simulink model "Smart_City_QCar2_self_driving_stack"  (R2024b)
settings: Solver=ode1  StartTime=0.0  StopTime=inf  FixedStep=Controller_Sample_Time  RelTol=1e-3  EnableMultiTasking=on
values from neighbouring files (symbols this model uses):
  angles_qcar2 = angles_new_qcar2(2: length (angles_new_qcar2), width (angles_new_qcar2)-5)    [Setup_QCar1and2_params.m]
  Audio_Sample_Time = 0.3    [Setup_QCar1and2_params.m]
  cal_pos = [0, 0, 0]    [Setup_QCar1and2_params.m]
  cameraStepSize = 3e-2    (= 0.03)    [Setup_QCar1and2_params.m]
  Cobra_Start = [0 0 0 0 0 0 0 0 0 0 0 0 ... (192000 elements, 192000x1)]    [QCar_Sounds.mat]
  Controller_Sample_Time = CSI_Sample_Time/10    (= 0.00166666666667)    [Setup_QCar1and2_params.m]
  CSI_Sample_Time = 1/60    (= 0.0166666666667)    [Setup_QCar1and2_params.m]
  engine = [0.455749511719 0.619506835938 0.612854003906 0.499603271484 0.347473144531 0.278045654297 0.304656982422 0.258544921875 0.100128173828 0.0902099609375 0.341461181641 0.515716552734 ... (88200 elements, 44100x2)]    [QCar_Sounds.mat]
  GyroKF_P0 = eye(2)    [Setup_QCar1and2_params.m]
  GyroKF_Q = diag([0.01, 0.001])    [Setup_QCar1and2_params.m]
  GyroKF_R = 0.01    [Setup_QCar1and2_params.m]
  GyroKF_X0 = [0;0]    [Setup_QCar1and2_params.m]
  honk = [0.01708984375 0.0179443359375 0.018798828125 0.019775390625 0.0209655761719 0.0218505859375 0.0221557617188 0.0223693847656 0.022705078125 0.023681640625 0.0252075195312 0.0257263183594 ... (43568 elements, 21784x2)]    [QCar_Sounds.mat]
  ImageDisplay_Sample_Time = CSI_Sample_Time*6    (= 0.1)    [Setup_QCar1and2_params.m]
  Initialization_Time = 5    [Setup_QCar1and2_params.m]
  LiDAR_Sample_Time = CSI_Sample_Time*3    (= 0.05)    [Setup_QCar1and2_params.m]
  map_mask = [1 1 1 0 0 1 0]    [Setup_QCar1and2_params.m]
  NN_Sample_Time = RealSense_Sample_Time*1    (= 0.0333333333333)    [Setup_QCar1and2_params.m]
  path_x = [0.826 0.836 0.846 0.856 0.866 0.876 0.886 0.896 0.906 0.916 0.926 0.936 ... (740 elements, 740x1)]    [SDCS_Paths_7.mat]
  path_x2 = [-0.614 -0.604 -0.594 -0.584 -0.574 -0.564 -0.554 -0.544 -0.534 -0.524 -0.514 -0.504 ... (1090 elements, 1090x1)]    [SDCS_Paths_7.mat]
  path_x3 = [-0.614 -0.603821428571 -0.593642857143 -0.583464285714 -0.573285714286 -0.563107142857 -0.552928571429 -0.54275 -0.532571428571 -0.522392857143 -0.512214285714 -0.502035714286 ... (714 elements, 714x1)]    [SDCS_Paths_7.mat]
  path_x4 = [-0.614 -0.604 -0.594 -0.584 -0.574 -0.564 -0.554 -0.544 -0.534 -0.524 -0.514 -0.504 ... (1761 elements, 1761x1)]    [SDCS_Paths_7.mat]
  path_x5 = [1.436 1.42588571429 1.41577142857 1.40565714286 1.39554285714 1.38542857143 1.37531428571 1.3652 1.35508571429 1.34497142857 1.33485714286 1.32474285714 ... (574 elements, 574x1)]    [SDCS_Paths_7.mat]
  path_x6 = [1.436 1.42588571429 1.41577142857 1.40565714286 1.39554285714 1.38542857143 1.37531428571 1.3652 1.35508571429 1.34497142857 1.33485714286 1.32474285714 ... (1288 elements, 1288x1)]    [SDCS_Paths_7.mat]
  path_x7 = [-1.5778487585 -1.56959877056 -1.56127865467 -1.55288878259 -1.54442952915 -1.53590127231 -1.52730439309 -1.51863927561 -1.50990630701 -1.50110587746 -1.49223838016 -1.4833042113 ... (2260 elements, 2260x1)]    [SDCS_Paths_7.mat]
  path_y = [-1.0887 -1.0887 -1.0887 -1.0887 -1.0887 -1.0887 -1.0887 -1.0887 -1.0887 -1.0887 -1.0887 -1.0887 ... (740 elements, 740x1)]    [SDCS_Paths_7.mat]
  path_y2 = [-1.0887 -1.0887 -1.0887 -1.0887 -1.0887 -1.0887 -1.0887 -1.0887 -1.0887 -1.0887 -1.0887 -1.0887 ... (1090 elements, 1090x1)]    [SDCS_Paths_7.mat]
  path_y3 = [-1.0887 -1.0887 -1.0887 -1.0887 -1.0887 -1.0887 -1.0887 -1.0887 -1.0887 -1.0887 -1.0887 -1.0887 ... (714 elements, 714x1)]    [SDCS_Paths_7.mat]
  path_y4 = [-1.0887 -1.0887 -1.0887 -1.0887 -1.0887 -1.0887 -1.0887 -1.0887 -1.0887 -1.0887 -1.0887 -1.0887 ... (1761 elements, 1761x1)]    [SDCS_Paths_7.mat]
  path_y5 = [-0.8157 -0.8157 -0.8157 -0.8157 -0.8157 -0.8157 -0.8157 -0.8157 -0.8157 -0.8157 -0.8157 -0.8157 ... (574 elements, 574x1)]    [SDCS_Paths_7.mat]
  path_y6 = [-0.8157 -0.8157 -0.8157 -0.8157 -0.8157 -0.8157 -0.8157 -0.8157 -0.8157 -0.8157 -0.8157 -0.8157 ... (1288 elements, 1288x1)]    [SDCS_Paths_7.mat]
  path_y7 = [-0.614490295955 -0.61974988896 -0.624981792226 -0.630185771997 -0.635361595765 -0.640509032279 -0.645627851559 -0.6507178249 -0.655778724888 -0.660810325409 -0.665812401655 -0.670784730139 ... (2260 elements, 2260x1)]    [SDCS_Paths_7.mat]
  put_me_down = [0 0 0 0 0 0 0 0 0 0 0 0 ... (335870 elements, 167935x2)]    [QCar_Sounds.mat]
  qcar2_lidar_to_map_rotation = 0    [Setup_QCar1and2_params.m]
  QCarEKF_L = 0.24    [Setup_QCar1and2_params.m]
  QCarEKF_P0 = eye(3)    [Setup_QCar1and2_params.m]
  QCarEKF_Q = diag([0.00001, 0.00001, 0.00001])    [Setup_QCar1and2_params.m]
  QCarEKF_R_combined = diag([0.1, 0.1, 0.01])    [Setup_QCar1and2_params.m]
  QCarEKF_R_heading = diag(0.1)    [Setup_QCar1and2_params.m]
  QcarKF_X0 = [0; 0; 0]    [Setup_QCar1and2_params.m]
  range_qcar2 = distance_new_qcar2(2: length (distance_new_qcar2), width (distance_new_qcar2)-5)    [Setup_QCar1and2_params.m]
  RealSense_Sample_Time = CSI_Sample_Time*2    (= 0.0333333333333)    [Setup_QCar1and2_params.m]
  truck_start = [0.00137329101562 0.00115966796875 0.0006103515625 0.000762939453125 0.00115966796875 0.00198364257812 0.00115966796875 0.000762939453125 0.00137329101562 0.00115966796875 0.00115966796875 0.000762939453125 ... (60000 elements, 60000x1)]    [QCar_Sounds.mat]
undefined symbols (not defined in the file or in its folder): DiscIntNeverNeededParam, gcbh, height, HIL, Joystick_Sample_Time, JPEG, left, Point, qc_get_step_size, top, video_display_show, width
libraries: quarc_library x65, simulink_extras x12, simulink x8
(part 3 of 5)

== system Smart_City_QCar2_self_driving_stack/QCar 2/QCar Control/QCar I//O ==
  note: '-w -d /tmp -uri %u', 'tcpip://192.168.1.3:17002'
  note: Command Conditioning
  note: HIL I/O
  note: LEDs:
      | 1. Back Left Amber
      | 2. Back Right Amber
      | 3. Front Left Amber
      | 4. Front Right Amber
      | 5. Brake Lights Red
      | 6. Reverse White
      | 7. Left Headlamps White
      | 8. Right Headlamps White
  "motorCmd (%, rad) [2]" : Inport
  Arm : Inport  Port=2
  Hazard : Inport  Port=3
  Volume : Inport  Port=4
  Honk : Inport  Port=5
  Abs : Abs  SaturateOnIntegerOverflow=off
  Audio : Subsystem
  Constant1 : Constant
  Constant3 : Constant  Value=.05
  Constant4 : Constant  Value=.05
  Constant6 : Constant  Value=2
  Demux : Demux  Outputs=2
  Display : Display
  Gain : Gain  Gain=+1
  Greater Than Threshold : Subsystem
  HIL Initialize : quarc_library/Data Acquisition/Generic/Configuration/HIL Initialize  object_name=HIL-1  board_type=qcar2  board_number=0  board_options=gyro_fs=250;gyro_rate=500;gyro_bw=125;gyro_ord=3;accel_fs=16;accel_rate=1000;accel_bw=250;accel_ord=3;temp_bw=4000;enc0_dir=0;enc1_dir=0;enc2_dir=0;steer_bias=0.05;  exclusive=off  active=on  hardware_clocks=[]  clock_modes=[]  initial_clock_frequencies=[]  set_clock_params_at_start=off  set_clock_params_at_switch_in=off  set_clock_frequencies_at_start=off  set_clock_frequencies_at_switch_in=off  analog_input_channels=[0:4]  analog_input_configurations=[]  analog_input_maximums=[3.3]  analog_input_minimums=[0]  set_analog_input_params_at_start=off  set_analog_input_params_at_switch_in=off  analog_output_channels=[]  analog_output_maximums=[]  analog_output_minimums=[]  initial_analog_outputs=[]  final_analog_outputs=[]  watchdog_analog_outputs=[]  set_analog_output_params_at_start=off  set_analog_output_params_at_switch_in=off  set_analog_outputs_at_start=off  set_analog_outputs_at_switch_in=off  set_analog_outputs_at_terminate=off  set_analog_outputs_at_switch_out=off  set_analog_outputs_on_watchdog=off  digital_input_channels=[0:14]  digital_output_channels=[11:26]  digital_output_configuration=[]  initial_digital_outputs=[0]  final_digital_outputs=[0]  watchdog_digital_outputs=[0]  set_digital_output_params_at_start=off  set_digital_output_params_at_switch_in=off  set_digital_outputs_at_start=on  set_digital_outputs_at_switch_in=off  set_digital_outputs_at_terminate=on  set_digital_outputs_at_switch_out=off  set_digital_outputs_on_watchdog=off  encoder_channels=[0:2]  quadrature=[4]  encoder_filter_frequency=100e6/1  initial_encoder_counts=[0]  set_encoder_params_at_start=on  set_encoder_params_at_switch_in=off  set_encoder_counts_at_start=on  set_encoder_counts_at_switch_in=off  pwm_channels=[0:1]  pwm_modes=[0]  pwm_frequency=180e6/4096  pwm_configuration=[0]  pwm_alignment=[0]  pwm_polarity=[1]  pwm_leading_deadband=[]  pwm_trailing_deadband=[]  initial_pwm_outputs=[0]  final_pwm_outputs=[0]  watchdog_pwm_outputs=[0]  set_pwm_params_at_start=on  set_pwm_params_at_switch_in=off  set_pwm_outputs_at_start=on  set_pwm_outputs_at_switch_in=off  set_pwm_outputs_at_terminate=on  set_pwm_outputs_at_switch_out=off  set_pwm_outputs_on_watchdog=off  other_output_channels=[1000 11000]  initial_other_outputs=[0]  final_other_outputs=[0]  watchdog_other_outputs=[0]  set_other_outputs_at_start=on  set_other_outputs_at_switch_in=off  set_other_outputs_at_terminate=on  set_other_outputs_at_switch_out=off  set_other_outputs_on_watchdog=off
  HIL Read : quarc_library/Data Acquisition/Generic/Immediate I//O/HIL Read  object_name=HIL-1  analog_channels=[4 2]  encoder_channels=[0]  digital_channels=[]  other_channels=[14000 3002 4001]  sample_time=qc_get_step_size  active=on  vector_output=off  data_type_mode=Inherit via back propagation  encoder_data_type=double  digital_data_type=boolean
  HIL Write : quarc_library/Data Acquisition/Generic/Immediate I//O/HIL Write  object_name=HIL-1  analog_channels=[]  pwm_channels=[]  digital_channels=[17:18 25:26 11:16 19:24]  other_channels=[1000 11000]  sample_time=-1  active=off  vector_input=on
  LEDs : Subsystem
  Less Than Threshold1 : Subsystem
  MATLAB Function : MATLAB Function  TreatAsAtomicUnit=on
  Memory : Memory
  Mux : Mux  Inputs=2
  Scope : Scope
  Steering Bias : Bias  Bias=0.05*-1  SaturateOnIntegerOverflow=off
  Unwrap 2^24 : quarc_library/Discontinuities/Inverse Modulus  modulus=16777215  output_derivative=off  output_revolutions=off  max_x=Inf  min_x=-Inf
  basicSpeedEstimation : Subsystem
  basicSpeedEstimation1 : Subsystem
  command saturation : Saturate  UpperLimit=.6  LowerLimit=-0.6
  direction convention : Gain  Gain=+1
  motorCurrent (A) [1] : Outport  VectorParamsAs1DForOutWhenUnconnected=off
  batteryVoltage (V) [1] : Outport  Port=2  VectorParamsAs1DForOutWhenUnconnected=off
  Speed (m/s) : Outport  Port=3  VectorParamsAs1DForOutWhenUnconnected=off
  gyroscopicRates (rad/s) : Outport  Port=4  VectorParamsAs1DForOutWhenUnconnected=off
  Odometer : Outport  Port=5  VectorParamsAs1DForOutWhenUnconnected=off
  wires:
  Demux/2 -> MATLAB Function/1(steering_in), LEDs/2(Steering)
  direction convention/1 -> command saturation/1
  "motorCmd (%, rad) [2]"/1 -> Demux/1
  HIL Read/3 -> Unwrap 2^24/1  "encoder counts"
  Gain/1 -> Steering Bias/1
  HIL Read/1 -> motorCurrent (A) [1]/1  "motor current"
  HIL Read/2 -> batteryVoltage (V) [1]/1  "battery voltage"
  HIL Read/4 -> basicSpeedEstimation/1(motorSpeed (counts/s))
  Unwrap 2^24/1 -> basicSpeedEstimation1/1(motorSpeed (counts/s))
  basicSpeedEstimation1/1(longitudinalCarSpeed (m/s)) -> Odometer/1
  basicSpeedEstimation/1(longitudinalCarSpeed (m/s)) -> [Speed], Speed (m/s)/1
  Demux/1 -> LEDs/1(Throttle), Scope/1, direction convention/1
  HIL Read/5 -> gyroscopicRates (rad/s)/1
  LEDs/1(LEDs) -> HIL Write/1
  Honk/1 -> Audio/1(Honk)
  Arm/1 -> Audio/2(Arm)
  [Speed] -> LEDs/3(Speed)
  Hazard/1 -> LEDs/4(Hazzard)
  HIL Read/6 -> Abs/1
  Abs/1 -> Greater Than Threshold/1(Signal)
  Constant6/1 -> Greater Than Threshold/2(Threshold)
  Constant1/1 -> Greater Than Threshold/3(Duration)
  Greater Than Threshold/1(elapsed) -> Audio/3(put_me_down)
  Volume/1 -> Audio/4(Volume)
  Constant3/1 -> Less Than Threshold1/2(Threshold)
  Constant4/1 -> Less Than Threshold1/3(Duration)
  [Speed] -> Less Than Threshold1/1(Signal)
  MATLAB Function/1(steering_out) -> Gain/1, Memory/1
  Less Than Threshold1/1(elapsed) -> Display/1, MATLAB Function/2(stopped)
  Memory/1 -> MATLAB Function/3(previous_steering)
  Mux/1 -> HIL Write/2
  Steering Bias/1 -> Mux/1
  command saturation/1 -> Mux/2

== system Smart_City_QCar2_self_driving_stack/QCar 2/QCar Control/bicycleModel ==
  note: coordinate transformation
  note: Model side slip angle beta
  note: steering servo dynamics
  heading (rad) : Inport
  "motorCommands (%, rad)" : Inport  Port=2
  carSpeed (m/s) : Inport  Port=3
  gyroscope (rad/s) : Inport  Port=4
  Add : Sum
  Divide : Product  Inputs=*/
  Lr : Constant  Value=0.128
  Mux3 : Mux  Inputs=3
  Product : Product
  Product1 : Product
  Product2 : Product
  Transfer Fcn : TransferFcn  Denominator=[0.1026 1]
  Trigonometric Function : Trigonometry
  Trigonometric Function1 : Trigonometry  Operator=cos
  Trigonometric Function2 : Trigonometry  Operator=tan
  Trigonometric Function3 : Trigonometry  Operator=atan
  select steering : Selector  InputPortWidth=2  IndexOptions=Index vector (dialog)  Indices=[2]  OutputSizes=1
  steering servo dynamics : Scope  NumInputPorts=2
  wheelbase : Constant  Value=0.256
  "poseRate (m/s, m/s, rad/s)" : Outport  VectorParamsAs1DForOutWhenUnconnected=off
  wires:
  Add/1 -> Trigonometric Function1/1, Trigonometric Function/1
  Trigonometric Function1/1 -> Product1/2
  Product/1 -> Mux3/2  "y_dot"
  select steering/1 -> Transfer Fcn/1, steering servo dynamics/1  "delta"
  carSpeed (m/s)/1 -> Product/2, Product1/1  "v"
  Product1/1 -> Mux3/1  "x_dot"
  Trigonometric Function/1 -> Product/1
  gyroscope (rad/s)/1 -> Mux3/3  "psi_dot"
  heading (rad)/1 -> Add/1  "psi"
  "motorCommands (%, rad)"/1 -> select steering/1
  Mux3/1 -> "poseRate (m/s, m/s, rad/s)"/1
  Transfer Fcn/1 -> Trigonometric Function2/1, steering servo dynamics/2
  Divide/1 -> Trigonometric Function3/1
  wheelbase/1 -> Divide/2
  Product2/1 -> Divide/1  "Lr tan(delta)"
  Trigonometric Function3/1 -> Add/2  "beta"
  Trigonometric Function2/1 -> Product2/1  "tan(delta)"
  Lr/1 -> Product2/2  "Lr"

== system Smart_City_QCar2_self_driving_stack/QCar 2/QCar Control/powerConsumptionMonitor ==
  note: Battery percentage calculation
  note: P = VI
  note: Electrical
      | power
      | consumed
  note: Power Monitoring Module:
      |
      | This subsystem monitors power consumption and provides a percentage battery remaining indicator.
      |
      | Inputs:
      | motorCurrent (A) n/a : Motor current being pulled by the main drive motor
      | batteryVoltage (V) {0, 12.6} : Current battery voltage reading
      |
      | Outputs:
      | motorPowerConsumption (W) n/a : Current power in Watts being pulled by the main drive motor
      | batteryLevel (%) {0,1} : Percentage battery level remaining
      |
      | Usage:
      | This is based on a maximum 3S battery voltage of 12.6 V (4.2V per cell) and minimum of 10.5 V (3.5V per cell)
  motorCurrent (A) [1] : Inport
  batteryVoltage (V) [1] : Inport  Port=2
  Divide : Product  Inputs=*/
  Gain : Gain  Gain=100
  Product : Product
  Subtract : Sum  Inputs=+-
  Subtract1 : Sum  Inputs=+-
  max voltage : Constant  Value=12.6
  min voltage : Constant  Value=10.5
  motorPowerConsumption (W) [1] : Outport  VectorParamsAs1DForOutWhenUnconnected=off
  batteryLevel (%) [1] : Outport  Port=2  VectorParamsAs1DForOutWhenUnconnected=off
  wires:
  Divide/1 -> Gain/1
  Subtract1/1 -> Divide/2
  Gain/1 -> batteryLevel (%) [1]/1
  Product/1 -> motorPowerConsumption (W) [1]/1
  min voltage/1 -> Subtract/2, Subtract1/2
  motorCurrent (A) [1]/1 -> Product/1
  max voltage/1 -> Subtract1/1
  Subtract/1 -> Divide/1
  batteryVoltage (V) [1]/1 -> Subtract/1, Product/2

== system Smart_City_QCar2_self_driving_stack/QCar 2/QCar Control/speedController ==
  note: Feedforward
  note: Feedback
  arm (0,1) : Inport
  desiredSpeed (m/s) : Inport  Port=2
  measuredSpeed (m/s) : Inport  Port=3
  Add : Sum
  Add1 : Sum
  Compare To Zero : simulink/Logic and Bit Operations/Compare To Zero  relop===  OutDataTypeStr=boolean
  Demux : Demux  Outputs=2
  Integrator1 : Integrator  ExternalReset=either  LimitOutput=on  UpperSaturationLimit=0.4  LowerSaturationLimit=-0.4
  Kff (% / m/s) : Gain  Gain=0.1
  "Ki (% / m) " : Gain
  Kp (% / m/s) : Gain  Gain=.3
  Multiply : Product
  Multiply1 : Product
  Multiply2 : Product
  Mux : Mux  Inputs=2
  Speed_Tracking : Scope  NumInputPorts=2
  Sum : Sum  Inputs=|+-
  command saturation : Saturate  UpperLimit=5  LowerLimit=-5
  throttleCmd (%) : Outport  VectorParamsAs1DForOutWhenUnconnected=off
  wires:
  command saturation/1 -> Multiply1/1  "desired"
  arm (0,1)/1 -> Multiply1/2, Multiply/2, Multiply2/2
  measuredSpeed (m/s)/1 -> Multiply/1  "meas"
  Multiply/1 -> Sum/2, Speed_Tracking/2  "measured"
  Add/1 -> Add1/2
  Add1/1 -> Multiply2/1  "%"
  Multiply1/1 -> Compare To Zero/1, Sum/1, Kff (% / m/s)/1, Speed_Tracking/1  "desired"
  Integrator1/1 -> Add/2
  Kp (% / m/s)/1 -> Add/1
  Compare To Zero/1 -> Integrator1/2
  Kff (% / m/s)/1 -> Add1/1
  Sum/1 -> "Ki (% / m) "/1, Kp (% / m/s)/1
  "Ki (% / m) "/1 -> Integrator1/1
  Multiply2/1 -> Mux/1  "pwm duty cycle"
  Mux/1 -> throttleCmd (%)/1
  desiredSpeed (m/s)/1 -> Demux/1
  Demux/1 -> command saturation/1
  Demux/2 -> Mux/2

== system Smart_City_QCar2_self_driving_stack/QCar 2/QCar Control/turnSpeedHandling ==
  Commands in : Inport
  Cos ^ : Inport  Port=2
  Cos : Trigonometry  Operator=cos
  Demux1 : Demux  Outputs=2
  Mux : Mux  Inputs=2
  Product : Product
  Saturation : Saturate  UpperLimit=1  LowerLimit=.3
  Speed Comparison : Scope  NumInputPorts=2
  Square : Math  Operator=pow  SignedPower=on
  Commands : Outport  VectorParamsAs1DForOutWhenUnconnected=off
  wires:
  Cos/1 -> Square/1
  Saturation/1 -> Product/2
  Demux1/1 -> Product/1, Speed Comparison/1  "Input Speed"
  Commands in/1 -> Demux1/1
  Cos ^/1 -> Square/2
  Square/1 -> Saturation/1
  Product/1 -> Mux/1, Speed Comparison/2  "Ouput Speed"
  Mux/1 -> Commands/1
  Demux1/2 -> Mux/2, Cos/1  "input steering"

== system Smart_City_QCar2_self_driving_stack/Randomizer1/Subsystem1/RisingEdge ==
  Input : Inport
  Logical Operator1 : Logic  AllPortsSameDT=off
  Logical Operator2 : Logic  Operator=NOT  AllPortsSameDT=off
  Memory : Memory  InheritSampleTime=on  LinearizeMemory=on
  RisingEdgeTrigger : Outport  VectorParamsAs1DForOutWhenUnconnected=off
  wires:
  Logical Operator1/1 -> RisingEdgeTrigger/1
  Logical Operator2/1 -> Logical Operator1/2
  Memory/1 -> Logical Operator2/1
  Input/1 -> Logical Operator1/1, Memory/1

== system Smart_City_QCar2_self_driving_stack/Speed & Steering Commander/Path Commander/Less Than Threshold ==
  note: Calculate Duration that Car is in Distance of Viable Path
  Distances : Inport
  Distance Threshold : Inport  Port=2
  Duration Threshold : Inport  Port=3
  Data Type Conversion : DataTypeConversion  SaturateOnIntegerOverflow=off  RndMeth=Floor
  Discrete-Time Integrator : DiscreteIntegrator  Priority=1  ExternalReset=level  SampleTime=qc_get_step_size  ICPrevOutput=DiscIntNeverNeededParam  ICPrevScaledInput=DiscIntNeverNeededParam
  Relational Operator : RelationalOperator  Operator=<  InputSameDT=off
  Relational Operator1 : RelationalOperator  InputSameDT=off
  Reset Condition : Logic  Operator=NOT  AllPortsSameDT=off  OutDataTypeStr=boolean
  elapsed : Outport  VectorParamsAs1DForOutWhenUnconnected=off
  wires:
  Data Type Conversion/1 -> Discrete-Time Integrator/1
  Distances/1 -> Relational Operator/1
  Distance Threshold/1 -> Relational Operator/2
  Relational Operator/1 -> Data Type Conversion/1, Reset Condition/1
  Reset Condition/1 -> Discrete-Time Integrator/2
  Discrete-Time Integrator/1 -> Relational Operator1/1
  Duration Threshold/1 -> Relational Operator1/2
  Relational Operator1/1 -> elapsed/1

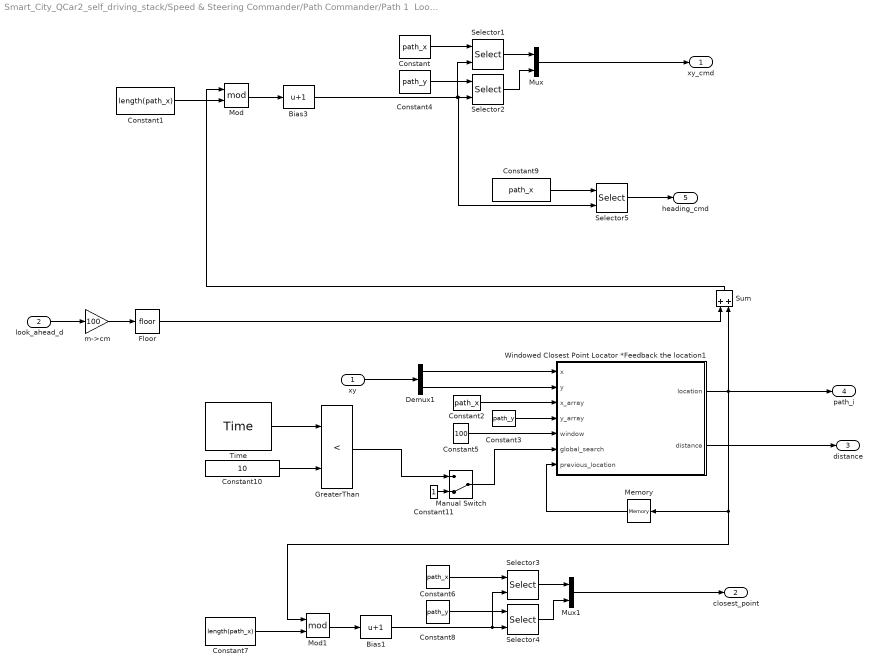
== system Smart_City_QCar2_self_driving_stack/Speed & Steering Commander/Path Commander/Path 1  Look Ahead Generator ==
  xy : Inport
  look_ahead_d : Inport  Port=2
  Bias1 : Bias  Bias=1  SaturateOnIntegerOverflow=off
  Bias3 : Bias  Bias=1  SaturateOnIntegerOverflow=off
  Constant{,2,6,9} (4 alike) : Constant  Value=path_x
  Constant1 : Constant  Value=length(path_x)
  Constant10 : Constant  Value=10
  Constant11 : Constant
  Constant3 : Constant  Value=path_y
  Constant4 : Constant  Value=path_y
  Constant5 : Constant  Value=100
  Constant7 : Constant  Value=length(path_x)
  Constant8 : Constant  Value=path_y
  Demux1 : Demux  Outputs=2
  Floor : Rounding
  GreaterThan : RelationalOperator  Operator=<  OutDataTypeStr=boolean  RndMeth=Simplest  InputSameDT=off
  Manual Switch : ManualSwitch  CurrentSetting=0
  Memory : Memory  InitialCondition=1  InheritSampleTime=on  LinearizeMemory=on  LinearizeAsDelay=on
  Mod : Math  Operator=mod
  Mod1 : Math  Operator=mod
  Mux : Mux  Inputs=2
  Mux1 : Mux  Inputs=2
  Selector{1..5} (5 alike) : Selector  InputPortWidth=length(path_x)  IndexOptions=Index vector (port)  Indices=[1 3]  OutputSizes=1
  Sum : Sum
  Time : quarc_library/Sources/Time/Time  time_source=Wall clock  sample_time=qc_get_step_size
  Windowed Closest Point Locator *Feedback the location1 : MATLAB Function  TreatAsAtomicUnit=on
  m->cm : Gain  Gain=100
  xy_cmd : Outport
  closest_point : Outport  Port=2
  distance : Outport  Port=3
  path_i : Outport  Port=4
  heading_cmd : Outport  Port=5
  wires:
  Demux1/1 -> Windowed Closest Point Locator *Feedback the location1/1(x)
  Constant2/1 -> Windowed Closest Point Locator *Feedback the location1/3(x_array)
  Constant3/1 -> Windowed Closest Point Locator *Feedback the location1/4(y_array)
  Constant1/1 -> Mod/2
  Sum/1 -> Mod/1
  Demux1/2 -> Windowed Closest Point Locator *Feedback the location1/2(y)
  Mod/1 -> Bias3/1
  xy/1 -> Demux1/1
  look_ahead_d/1 -> m->cm/1
  m->cm/1 -> Floor/1
  Floor/1 -> Sum/1
  Constant/1 -> Selector1/1
  Selector1/1 -> Mux/1
  Constant4/1 -> Selector2/1
  Mux/1 -> xy_cmd/1
  Selector2/1 -> Mux/2
  Windowed Closest Point Locator *Feedback the location1/2(distance) -> distance/1
  Mux1/1 -> closest_point/1
  Bias1/1 -> Selector3/2, Selector4/2
  Selector4/1 -> Mux1/2
  Constant6/1 -> Selector3/1
  Mod1/1 -> Bias1/1
  Constant7/1 -> Mod1/2
  Constant8/1 -> Selector4/1
  Selector3/1 -> Mux1/1
  Windowed Closest Point Locator *Feedback the location1/1(location) -> Sum/2, path_i/1, Mod1/1, Memory/1
  Bias3/1 -> Selector1/2, Selector5/2, Selector2/2
  Constant9/1 -> Selector5/1
  Selector5/1 -> heading_cmd/1
  Time/1 -> GreaterThan/1
  Constant10/1 -> GreaterThan/2
  Constant5/1 -> Windowed Closest Point Locator *Feedback the location1/5(window)
  Memory/1 -> Windowed Closest Point Locator *Feedback the location1/7(previous_location)
  Constant11/1 -> Manual Switch/2
  Manual Switch/1 -> Windowed Closest Point Locator *Feedback the location1/6(global_search)
  GreaterThan/1 -> Manual Switch/1

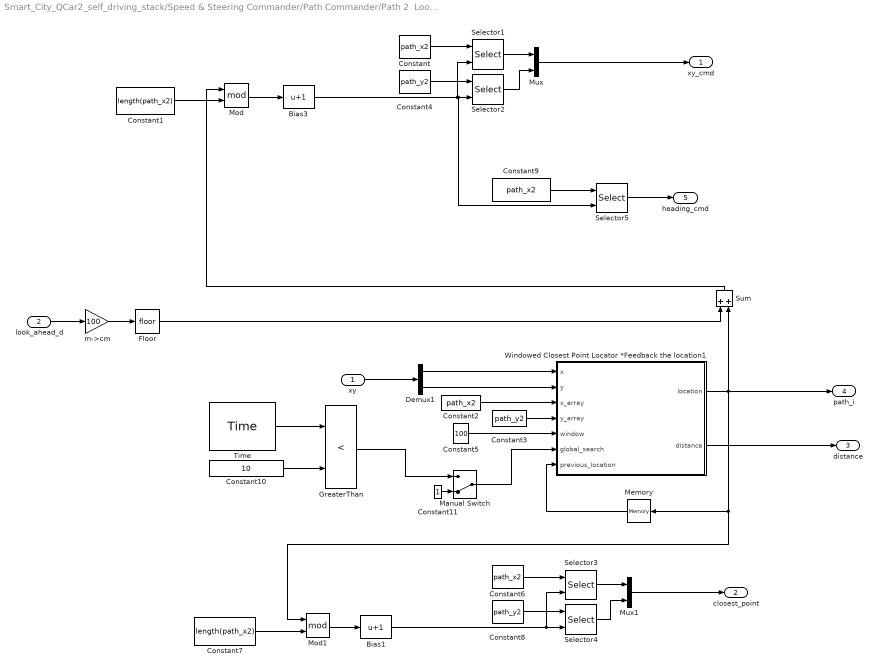
== system Smart_City_QCar2_self_driving_stack/Speed & Steering Commander/Path Commander/Path 2  Look Ahead Generator ==
  xy : Inport
  look_ahead_d : Inport  Port=2
  Bias1 : Bias  Bias=1  SaturateOnIntegerOverflow=off
  Bias3 : Bias  Bias=1  SaturateOnIntegerOverflow=off
  Constant{,2,6,9} (4 alike) : Constant  Value=path_x2
  Constant1 : Constant  Value=length(path_x2)
  Constant10 : Constant  Value=10
  Constant11 : Constant
  Constant3 : Constant  Value=path_y2
  Constant4 : Constant  Value=path_y2
  Constant5 : Constant  Value=100
  Constant7 : Constant  Value=length(path_x2)
  Constant8 : Constant  Value=path_y2
  Demux1 : Demux  Outputs=2
  Floor : Rounding
  GreaterThan : RelationalOperator  Operator=<  OutDataTypeStr=boolean  RndMeth=Simplest  InputSameDT=off
  Manual Switch : ManualSwitch  CurrentSetting=0
  Memory : Memory  InitialCondition=1  InheritSampleTime=on  LinearizeMemory=on  LinearizeAsDelay=on
  Mod : Math  Operator=mod
  Mod1 : Math  Operator=mod
  Mux : Mux  Inputs=2
  Mux1 : Mux  Inputs=2
  Selector{1..5} (5 alike) : Selector  InputPortWidth=length(path_x2)  IndexOptions=Index vector (port)  Indices=[1 3]  OutputSizes=1
  Sum : Sum
  Time : quarc_library/Sources/Time/Time  time_source=Wall clock  sample_time=qc_get_step_size
  Windowed Closest Point Locator *Feedback the location1 : MATLAB Function  TreatAsAtomicUnit=on
  m->cm : Gain  Gain=100
  xy_cmd : Outport
  closest_point : Outport  Port=2
  distance : Outport  Port=3
  path_i : Outport  Port=4
  heading_cmd : Outport  Port=5
  wires:
  Memory/1 -> Windowed Closest Point Locator *Feedback the location1/7(previous_location)
  Constant5/1 -> Windowed Closest Point Locator *Feedback the location1/5(window)
  Selector5/1 -> heading_cmd/1
  Constant9/1 -> Selector5/1
  Bias3/1 -> Selector2/2, Selector5/2, Selector1/2
  Windowed Closest Point Locator *Feedback the location1/1(location) -> Memory/1, Mod1/1, path_i/1, Sum/2
  Constant7/1 -> Mod1/2
  Mod1/1 -> Bias1/1
  Windowed Closest Point Locator *Feedback the location1/2(distance) -> distance/1
  Selector2/1 -> Mux/2
  Mux/1 -> xy_cmd/1
  Constant4/1 -> Selector2/1
  Selector1/1 -> Mux/1
  Constant/1 -> Selector1/1
  Floor/1 -> Sum/1
  m->cm/1 -> Floor/1
  look_ahead_d/1 -> m->cm/1
  xy/1 -> Demux1/1
  Mod/1 -> Bias3/1
  Demux1/2 -> Windowed Closest Point Locator *Feedback the location1/2(y)
  Sum/1 -> Mod/1
  Constant1/1 -> Mod/2
  Constant3/1 -> Windowed Closest Point Locator *Feedback the location1/4(y_array)
  Constant2/1 -> Windowed Closest Point Locator *Feedback the location1/3(x_array)
  Demux1/1 -> Windowed Closest Point Locator *Feedback the location1/1(x)
  Constant8/1 -> Selector4/1
  Selector3/1 -> Mux1/1
  Constant6/1 -> Selector3/1
  Bias1/1 -> Selector3/2, Selector4/2
  Selector4/1 -> Mux1/2
  Mux1/1 -> closest_point/1
  Time/1 -> GreaterThan/1
  Constant10/1 -> GreaterThan/2
  Manual Switch/1 -> Windowed Closest Point Locator *Feedback the location1/6(global_search)
  Constant11/1 -> Manual Switch/2
  GreaterThan/1 -> Manual Switch/1

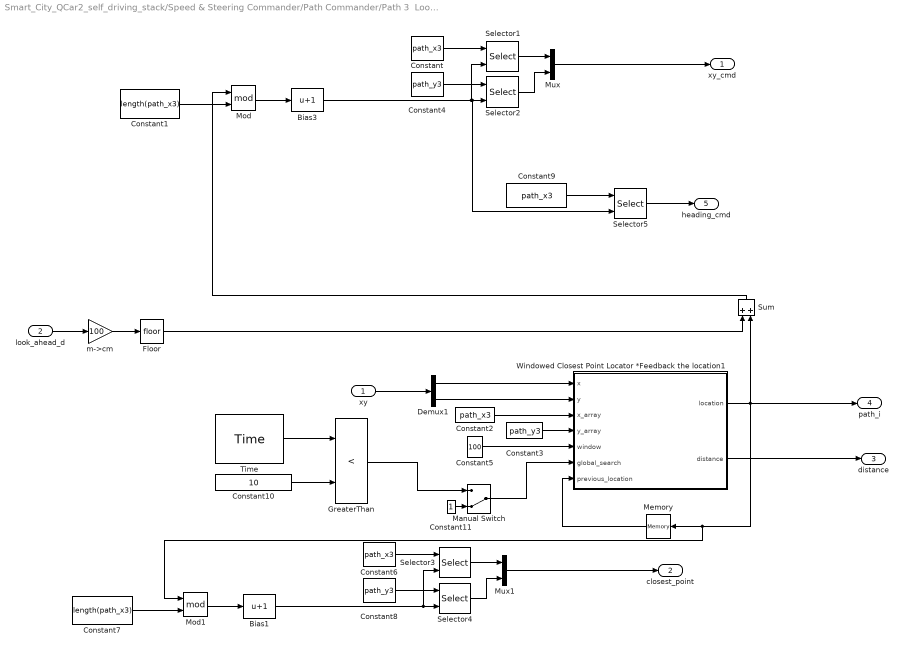
== system Smart_City_QCar2_self_driving_stack/Speed & Steering Commander/Path Commander/Path 3  Look Ahead Generator ==
  xy : Inport
  look_ahead_d : Inport  Port=2
  Bias1 : Bias  Bias=1  SaturateOnIntegerOverflow=off
  Bias3 : Bias  Bias=1  SaturateOnIntegerOverflow=off
  Constant{,2,6,9} (4 alike) : Constant  Value=path_x3
  Constant1 : Constant  Value=length(path_x3)
  Constant10 : Constant  Value=10
  Constant11 : Constant
  Constant3 : Constant  Value=path_y3
  Constant4 : Constant  Value=path_y3
  Constant5 : Constant  Value=100
  Constant7 : Constant  Value=length(path_x3)
  Constant8 : Constant  Value=path_y3
  Demux1 : Demux  Outputs=2
  Floor : Rounding
  GreaterThan : RelationalOperator  Operator=<  OutDataTypeStr=boolean  RndMeth=Simplest  InputSameDT=off
  Manual Switch : ManualSwitch  CurrentSetting=0
  Memory : Memory  InitialCondition=1  InheritSampleTime=on  LinearizeMemory=on  LinearizeAsDelay=on
  Mod : Math  Operator=mod
  Mod1 : Math  Operator=mod
  Mux : Mux  Inputs=2
  Mux1 : Mux  Inputs=2
  Selector{1..5} (5 alike) : Selector  InputPortWidth=length(path_x3)  IndexOptions=Index vector (port)  Indices=[1 3]  OutputSizes=1
  Sum : Sum
  Time : quarc_library/Sources/Time/Time  time_source=Wall clock  sample_time=qc_get_step_size
  Windowed Closest Point Locator *Feedback the location1 : MATLAB Function  TreatAsAtomicUnit=on
  m->cm : Gain  Gain=100
  xy_cmd : Outport
  closest_point : Outport  Port=2
  distance : Outport  Port=3
  path_i : Outport  Port=4
  heading_cmd : Outport  Port=5
  wires:
  Demux1/1 -> Windowed Closest Point Locator *Feedback the location1/1(x)
  Constant2/1 -> Windowed Closest Point Locator *Feedback the location1/3(x_array)
  Constant3/1 -> Windowed Closest Point Locator *Feedback the location1/4(y_array)
  Constant1/1 -> Mod/2
  Sum/1 -> Mod/1
  Demux1/2 -> Windowed Closest Point Locator *Feedback the location1/2(y)
  Mod/1 -> Bias3/1
  xy/1 -> Demux1/1
  look_ahead_d/1 -> m->cm/1
  m->cm/1 -> Floor/1
  Floor/1 -> Sum/1
  Constant/1 -> Selector1/1
  Selector1/1 -> Mux/1
  Constant4/1 -> Selector2/1
  Mux/1 -> xy_cmd/1
  Selector2/1 -> Mux/2
  Windowed Closest Point Locator *Feedback the location1/2(distance) -> distance/1
  Bias3/1 -> Selector1/2, Selector5/2, Selector2/2
  Constant9/1 -> Selector5/1
  Selector5/1 -> heading_cmd/1
  Constant5/1 -> Windowed Closest Point Locator *Feedback the location1/5(window)
  Memory/1 -> Windowed Closest Point Locator *Feedback the location1/7(previous_location)
  Selector4/1 -> Mux1/2
  Selector3/1 -> Mux1/1
  Mux1/1 -> closest_point/1
  Constant8/1 -> Selector4/1
  Windowed Closest Point Locator *Feedback the location1/1(location) -> Sum/2, path_i/1, Mod1/1, Memory/1
  Mod1/1 -> Bias1/1
  Constant6/1 -> Selector3/1
  Constant7/1 -> Mod1/2
  Bias1/1 -> Selector3/2, Selector4/2
  Time/1 -> GreaterThan/1
  Constant10/1 -> GreaterThan/2
  Manual Switch/1 -> Windowed Closest Point Locator *Feedback the location1/6(global_search)
  Constant11/1 -> Manual Switch/2
  GreaterThan/1 -> Manual Switch/1

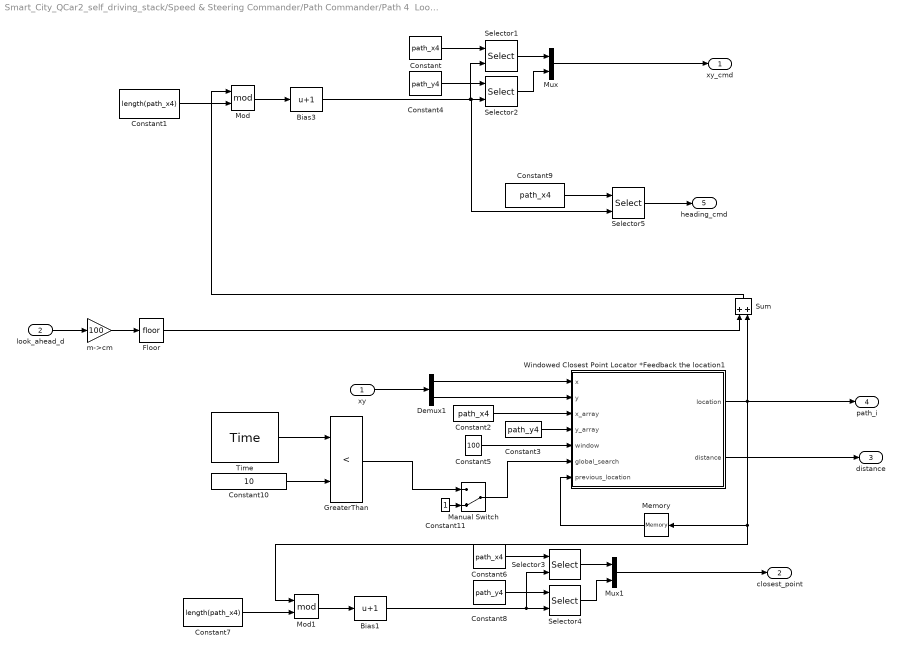
== system Smart_City_QCar2_self_driving_stack/Speed & Steering Commander/Path Commander/Path 4  Look Ahead Generator ==
  xy : Inport
  look_ahead_d : Inport  Port=2
  Bias1 : Bias  Bias=1  SaturateOnIntegerOverflow=off
  Bias3 : Bias  Bias=1  SaturateOnIntegerOverflow=off
  Constant{,2,6,9} (4 alike) : Constant  Value=path_x4
  Constant1 : Constant  Value=length(path_x4)
  Constant10 : Constant  Value=10
  Constant11 : Constant
  Constant3 : Constant  Value=path_y4
  Constant4 : Constant  Value=path_y4
  Constant5 : Constant  Value=100
  Constant7 : Constant  Value=length(path_x4)
  Constant8 : Constant  Value=path_y4
  Demux1 : Demux  Outputs=2
  Floor : Rounding
  GreaterThan : RelationalOperator  Operator=<  OutDataTypeStr=boolean  RndMeth=Simplest  InputSameDT=off
  Manual Switch : ManualSwitch  CurrentSetting=0
  Memory : Memory  InitialCondition=1  InheritSampleTime=on  LinearizeMemory=on  LinearizeAsDelay=on
  Mod : Math  Operator=mod
  Mod1 : Math  Operator=mod
  Mux : Mux  Inputs=2
  Mux1 : Mux  Inputs=2
  Selector{1..5} (5 alike) : Selector  InputPortWidth=length(path_x4)  IndexOptions=Index vector (port)  Indices=[1 3]  OutputSizes=1
  Sum : Sum
  Time : quarc_library/Sources/Time/Time  time_source=Wall clock  sample_time=qc_get_step_size
  Windowed Closest Point Locator *Feedback the location1 : MATLAB Function  TreatAsAtomicUnit=on
  m->cm : Gain  Gain=100
  xy_cmd : Outport
  closest_point : Outport  Port=2
  distance : Outport  Port=3
  path_i : Outport  Port=4
  heading_cmd : Outport  Port=5
  wires:
  Windowed Closest Point Locator *Feedback the location1/1(location) -> Mod1/1, Memory/1, path_i/1, Sum/2
  Memory/1 -> Windowed Closest Point Locator *Feedback the location1/7(previous_location)
  Constant5/1 -> Windowed Closest Point Locator *Feedback the location1/5(window)
  Selector5/1 -> heading_cmd/1
  Constant9/1 -> Selector5/1
  Bias3/1 -> Selector2/2, Selector5/2, Selector1/2
  Windowed Closest Point Locator *Feedback the location1/2(distance) -> distance/1
  Selector2/1 -> Mux/2
  Mux/1 -> xy_cmd/1
  Constant4/1 -> Selector2/1
  Selector1/1 -> Mux/1
  Constant/1 -> Selector1/1
  Floor/1 -> Sum/1
  m->cm/1 -> Floor/1
  look_ahead_d/1 -> m->cm/1
  xy/1 -> Demux1/1
  Mod/1 -> Bias3/1
  Demux1/2 -> Windowed Closest Point Locator *Feedback the location1/2(y)
  Sum/1 -> Mod/1
  Constant1/1 -> Mod/2
  Constant3/1 -> Windowed Closest Point Locator *Feedback the location1/4(y_array)
  Constant2/1 -> Windowed Closest Point Locator *Feedback the location1/3(x_array)
  Demux1/1 -> Windowed Closest Point Locator *Feedback the location1/1(x)
  Mux1/1 -> closest_point/1
  Mod1/1 -> Bias1/1
  Selector4/1 -> Mux1/2
  Constant7/1 -> Mod1/2
  Selector3/1 -> Mux1/1
  Constant8/1 -> Selector4/1
  Bias1/1 -> Selector3/2, Selector4/2
  Constant6/1 -> Selector3/1
  Time/1 -> GreaterThan/1
  Constant10/1 -> GreaterThan/2
  Manual Switch/1 -> Windowed Closest Point Locator *Feedback the location1/6(global_search)
  Constant11/1 -> Manual Switch/2
  GreaterThan/1 -> Manual Switch/1

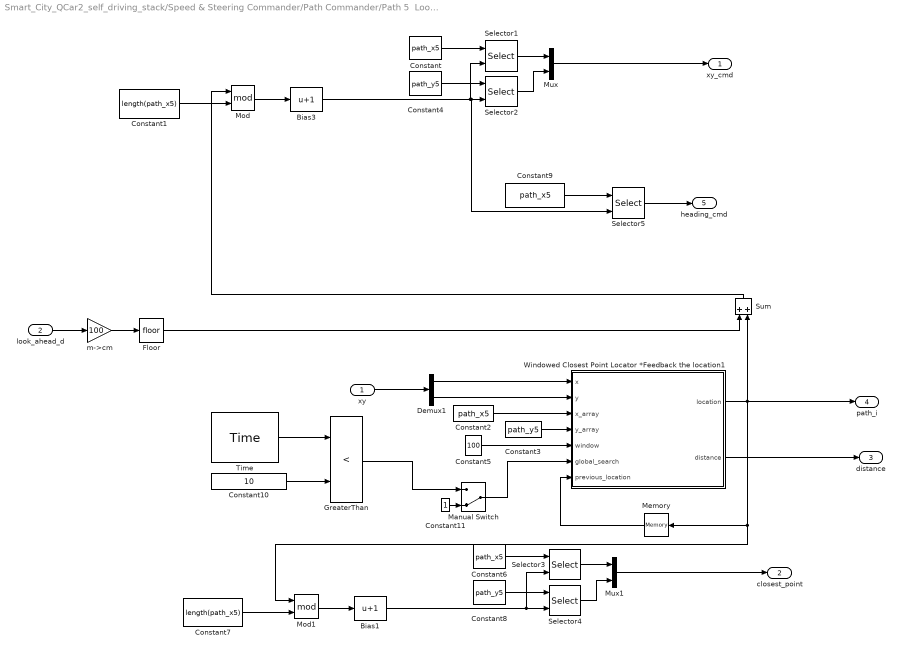
== system Smart_City_QCar2_self_driving_stack/Speed & Steering Commander/Path Commander/Path 5  Look Ahead Generator ==
  xy : Inport
  look_ahead_d : Inport  Port=2
  Bias1 : Bias  Bias=1  SaturateOnIntegerOverflow=off
  Bias3 : Bias  Bias=1  SaturateOnIntegerOverflow=off
  Constant{,2,6,9} (4 alike) : Constant  Value=path_x5
  Constant1 : Constant  Value=length(path_x5)
  Constant10 : Constant  Value=10
  Constant11 : Constant
  Constant3 : Constant  Value=path_y5
  Constant4 : Constant  Value=path_y5
  Constant5 : Constant  Value=100
  Constant7 : Constant  Value=length(path_x5)
  Constant8 : Constant  Value=path_y5
  Demux1 : Demux  Outputs=2
  Floor : Rounding
  GreaterThan : RelationalOperator  Operator=<  OutDataTypeStr=boolean  RndMeth=Simplest  InputSameDT=off
  Manual Switch : ManualSwitch  CurrentSetting=0
  Memory : Memory  InitialCondition=1  InheritSampleTime=on  LinearizeMemory=on  LinearizeAsDelay=on
  Mod : Math  Operator=mod
  Mod1 : Math  Operator=mod
  Mux : Mux  Inputs=2
  Mux1 : Mux  Inputs=2
  Selector{1..5} (5 alike) : Selector  InputPortWidth=length(path_x5)  IndexOptions=Index vector (port)  Indices=[1 3]  OutputSizes=1
  Sum : Sum
  Time : quarc_library/Sources/Time/Time  time_source=Wall clock  sample_time=qc_get_step_size
  Windowed Closest Point Locator *Feedback the location1 : MATLAB Function  TreatAsAtomicUnit=on
  m->cm : Gain  Gain=100
  xy_cmd : Outport
  closest_point : Outport  Port=2
  distance : Outport  Port=3
  path_i : Outport  Port=4
  heading_cmd : Outport  Port=5
  wires:
  GreaterThan/1 -> Manual Switch/1
  Constant11/1 -> Manual Switch/2
  Manual Switch/1 -> Windowed Closest Point Locator *Feedback the location1/6(global_search)
  Constant10/1 -> GreaterThan/2
  Time/1 -> GreaterThan/1
  Constant6/1 -> Selector3/1
  Bias1/1 -> Selector4/2, Selector3/2
  Constant8/1 -> Selector4/1
  Selector3/1 -> Mux1/1
  Constant7/1 -> Mod1/2
  Selector4/1 -> Mux1/2
  Mod1/1 -> Bias1/1
  Mux1/1 -> closest_point/1
  Demux1/1 -> Windowed Closest Point Locator *Feedback the location1/1(x)
  Constant2/1 -> Windowed Closest Point Locator *Feedback the location1/3(x_array)
  Constant3/1 -> Windowed Closest Point Locator *Feedback the location1/4(y_array)
  Constant1/1 -> Mod/2
  Sum/1 -> Mod/1
  Demux1/2 -> Windowed Closest Point Locator *Feedback the location1/2(y)
  Mod/1 -> Bias3/1
  xy/1 -> Demux1/1
  look_ahead_d/1 -> m->cm/1
  m->cm/1 -> Floor/1
  Floor/1 -> Sum/1
  Constant/1 -> Selector1/1
  Selector1/1 -> Mux/1
  Constant4/1 -> Selector2/1
  Mux/1 -> xy_cmd/1
  Selector2/1 -> Mux/2
  Windowed Closest Point Locator *Feedback the location1/2(distance) -> distance/1
  Bias3/1 -> Selector1/2, Selector5/2, Selector2/2
  Constant9/1 -> Selector5/1
  Selector5/1 -> heading_cmd/1
  Constant5/1 -> Windowed Closest Point Locator *Feedback the location1/5(window)
  Memory/1 -> Windowed Closest Point Locator *Feedback the location1/7(previous_location)
  Windowed Closest Point Locator *Feedback the location1/1(location) -> Sum/2, path_i/1, Memory/1, Mod1/1

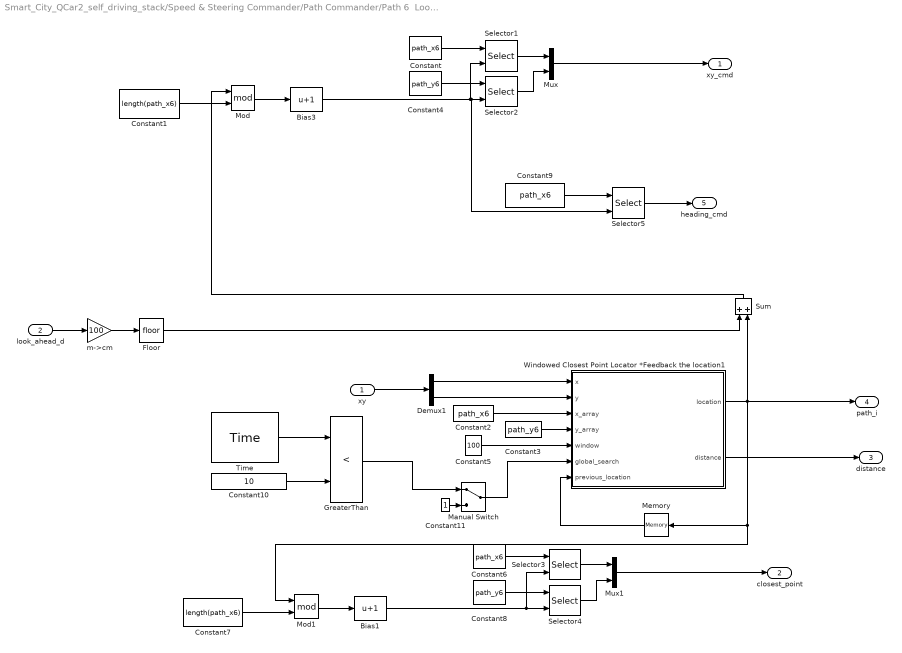
== system Smart_City_QCar2_self_driving_stack/Speed & Steering Commander/Path Commander/Path 6  Look Ahead Generator ==
  xy : Inport
  look_ahead_d : Inport  Port=2
  Bias1 : Bias  Bias=1  SaturateOnIntegerOverflow=off
  Bias3 : Bias  Bias=1  SaturateOnIntegerOverflow=off
  Constant{,2,6,9} (4 alike) : Constant  Value=path_x6
  Constant1 : Constant  Value=length(path_x6)
  Constant10 : Constant  Value=10
  Constant11 : Constant
  Constant3 : Constant  Value=path_y6
  Constant4 : Constant  Value=path_y6
  Constant5 : Constant  Value=100
  Constant7 : Constant  Value=length(path_x6)
  Constant8 : Constant  Value=path_y6
  Demux1 : Demux  Outputs=2
  Floor : Rounding
  GreaterThan : RelationalOperator  Operator=<  OutDataTypeStr=boolean  RndMeth=Simplest  InputSameDT=off
  Manual Switch : ManualSwitch
  Memory : Memory  InitialCondition=1  InheritSampleTime=on  LinearizeMemory=on  LinearizeAsDelay=on
  Mod : Math  Operator=mod
  Mod1 : Math  Operator=mod
  Mux : Mux  Inputs=2
  Mux1 : Mux  Inputs=2
  Selector{1..5} (5 alike) : Selector  InputPortWidth=length(path_x6)  IndexOptions=Index vector (port)  Indices=[1 3]  OutputSizes=1
  Sum : Sum
  Time : quarc_library/Sources/Time/Time  time_source=Wall clock  sample_time=qc_get_step_size
  Windowed Closest Point Locator *Feedback the location1 : MATLAB Function  TreatAsAtomicUnit=on
  m->cm : Gain  Gain=100
  xy_cmd : Outport
  closest_point : Outport  Port=2
  distance : Outport  Port=3
  path_i : Outport  Port=4
  heading_cmd : Outport  Port=5
  wires:
  Windowed Closest Point Locator *Feedback the location1/1(location) -> Mod1/1, Memory/1, path_i/1, Sum/2
  Memory/1 -> Windowed Closest Point Locator *Feedback the location1/7(previous_location)
  Constant5/1 -> Windowed Closest Point Locator *Feedback the location1/5(window)
  Selector5/1 -> heading_cmd/1
  Constant9/1 -> Selector5/1
  Bias3/1 -> Selector2/2, Selector5/2, Selector1/2
  Windowed Closest Point Locator *Feedback the location1/2(distance) -> distance/1
  Selector2/1 -> Mux/2
  Mux/1 -> xy_cmd/1
  Constant4/1 -> Selector2/1
  Selector1/1 -> Mux/1
  Constant/1 -> Selector1/1
  Floor/1 -> Sum/1
  m->cm/1 -> Floor/1
  look_ahead_d/1 -> m->cm/1
  xy/1 -> Demux1/1
  Mod/1 -> Bias3/1
  Demux1/2 -> Windowed Closest Point Locator *Feedback the location1/2(y)
  Sum/1 -> Mod/1
  Constant1/1 -> Mod/2
  Constant3/1 -> Windowed Closest Point Locator *Feedback the location1/4(y_array)
  Constant2/1 -> Windowed Closest Point Locator *Feedback the location1/3(x_array)
  Demux1/1 -> Windowed Closest Point Locator *Feedback the location1/1(x)
  Mux1/1 -> closest_point/1
  Mod1/1 -> Bias1/1
  Selector4/1 -> Mux1/2
  Constant7/1 -> Mod1/2
  Selector3/1 -> Mux1/1
  Constant8/1 -> Selector4/1
  Bias1/1 -> Selector3/2, Selector4/2
  Constant6/1 -> Selector3/1
  Time/1 -> GreaterThan/1
  Constant10/1 -> GreaterThan/2
  Manual Switch/1 -> Windowed Closest Point Locator *Feedback the location1/6(global_search)
  Constant11/1 -> Manual Switch/2
  GreaterThan/1 -> Manual Switch/1

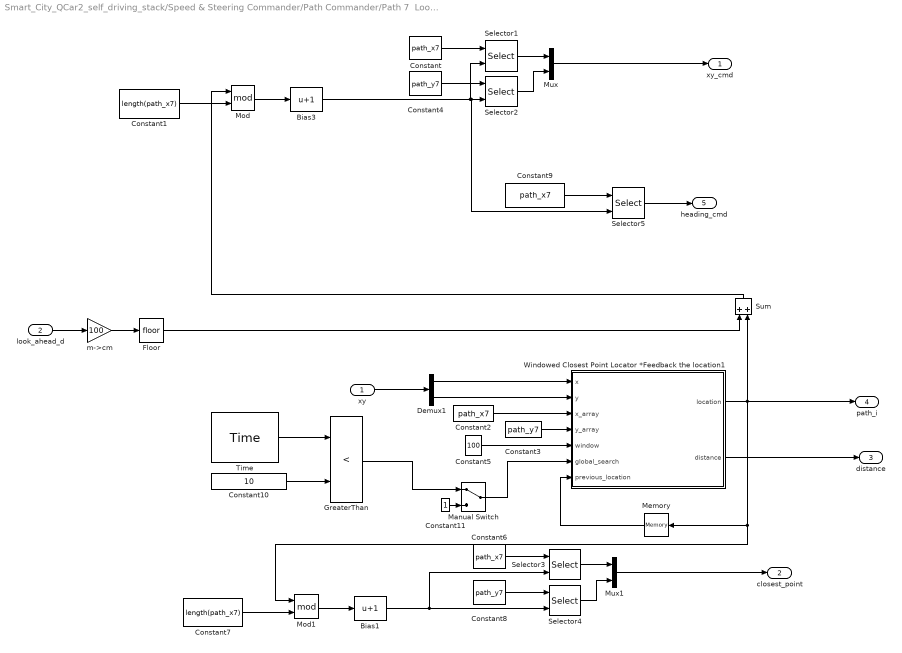
== system Smart_City_QCar2_self_driving_stack/Speed & Steering Commander/Path Commander/Path 7  Look Ahead Generator ==
  xy : Inport
  look_ahead_d : Inport  Port=2
  Bias1 : Bias  Bias=1  SaturateOnIntegerOverflow=off
  Bias3 : Bias  Bias=1  SaturateOnIntegerOverflow=off
  Constant{,2,6,9} (4 alike) : Constant  Value=path_x7
  Constant1 : Constant  Value=length(path_x7)
  Constant10 : Constant  Value=10
  Constant11 : Constant
  Constant3 : Constant  Value=path_y7
  Constant4 : Constant  Value=path_y7
  Constant5 : Constant  Value=100
  Constant7 : Constant  Value=length(path_x7)
  Constant8 : Constant  Value=path_y7
  Demux1 : Demux  Outputs=2
  Floor : Rounding
  GreaterThan : RelationalOperator  Operator=<  OutDataTypeStr=boolean  RndMeth=Simplest  InputSameDT=off
  Manual Switch : ManualSwitch
  Memory : Memory  InitialCondition=1  InheritSampleTime=on  LinearizeMemory=on  LinearizeAsDelay=on
  Mod : Math  Operator=mod
  Mod1 : Math  Operator=mod
  Mux : Mux  Inputs=2
  Mux1 : Mux  Inputs=2
  Selector{1..5} (5 alike) : Selector  InputPortWidth=length(path_x7)  IndexOptions=Index vector (port)  Indices=[1 3]  OutputSizes=1
  Sum : Sum
  Time : quarc_library/Sources/Time/Time  time_source=Wall clock  sample_time=qc_get_step_size
  Windowed Closest Point Locator *Feedback the location1 : MATLAB Function  TreatAsAtomicUnit=on
  m->cm : Gain  Gain=100
  xy_cmd : Outport
  closest_point : Outport  Port=2
  distance : Outport  Port=3
  path_i : Outport  Port=4
  heading_cmd : Outport  Port=5
  wires:
  Windowed Closest Point Locator *Feedback the location1/1(location) -> Mod1/1, Memory/1, path_i/1, Sum/2
  Memory/1 -> Windowed Closest Point Locator *Feedback the location1/7(previous_location)
  Constant5/1 -> Windowed Closest Point Locator *Feedback the location1/5(window)
  Selector5/1 -> heading_cmd/1
  Constant9/1 -> Selector5/1
  Bias3/1 -> Selector2/2, Selector5/2, Selector1/2
  Windowed Closest Point Locator *Feedback the location1/2(distance) -> distance/1
  Selector2/1 -> Mux/2
  Mux/1 -> xy_cmd/1
  Constant4/1 -> Selector2/1
  Selector1/1 -> Mux/1
  Constant/1 -> Selector1/1
  Floor/1 -> Sum/1
  m->cm/1 -> Floor/1
  look_ahead_d/1 -> m->cm/1
  xy/1 -> Demux1/1
  Mod/1 -> Bias3/1
  Demux1/2 -> Windowed Closest Point Locator *Feedback the location1/2(y)
  Sum/1 -> Mod/1
  Constant1/1 -> Mod/2
  Constant3/1 -> Windowed Closest Point Locator *Feedback the location1/4(y_array)
  Constant2/1 -> Windowed Closest Point Locator *Feedback the location1/3(x_array)
  Demux1/1 -> Windowed Closest Point Locator *Feedback the location1/1(x)
  Mux1/1 -> closest_point/1
  Mod1/1 -> Bias1/1
  Selector4/1 -> Mux1/2
  Constant7/1 -> Mod1/2
  Selector3/1 -> Mux1/1
  Constant8/1 -> Selector4/1
  Bias1/1 -> Selector3/2, Selector4/2
  Constant6/1 -> Selector3/1
  Time/1 -> GreaterThan/1
  Constant10/1 -> GreaterThan/2
  Manual Switch/1 -> Windowed Closest Point Locator *Feedback the location1/6(global_search)
  Constant11/1 -> Manual Switch/2
  GreaterThan/1 -> Manual Switch/1

== system Smart_City_QCar2_self_driving_stack/Speed & Steering Commander/Sign Finder/Greater Than Threshold ==
  Signal : Inport
  Threshold : Inport  Port=2
  Duration : Inport  Port=3
  Data Type Conversion : DataTypeConversion  SaturateOnIntegerOverflow=off  RndMeth=Floor
  Discrete-Time Integrator : DiscreteIntegrator  Priority=1  ExternalReset=level  SampleTime=qc_get_step_size  ICPrevOutput=DiscIntNeverNeededParam  ICPrevScaledInput=DiscIntNeverNeededParam
  Logical Operator : Logic  Operator=NOT  AllPortsSameDT=off  OutDataTypeStr=boolean
  Relational Operator : RelationalOperator  InputSameDT=off
  Relational Operator1 : RelationalOperator  InputSameDT=off
  elapsed : Outport  VectorParamsAs1DForOutWhenUnconnected=off
  time : Outport  Port=2  VectorParamsAs1DForOutWhenUnconnected=off
  wires:
  Relational Operator1/1 -> elapsed/1
  Duration/1 -> Relational Operator1/2
  Discrete-Time Integrator/1 -> time/1, Relational Operator1/1
  Logical Operator/1 -> Discrete-Time Integrator/2
  Relational Operator/1 -> Logical Operator/1, Data Type Conversion/1
  Threshold/1 -> Relational Operator/2
  Signal/1 -> Relational Operator/1
  Data Type Conversion/1 -> Discrete-Time Integrator/1

== system Smart_City_QCar2_self_driving_stack/Speed & Steering Commander/Sign Finder/Greater Than Threshold1 ==
  Signal : Inport
  Threshold : Inport  Port=2
  Duration : Inport  Port=3
  Data Type Conversion : DataTypeConversion  SaturateOnIntegerOverflow=off  RndMeth=Floor
  Discrete-Time Integrator : DiscreteIntegrator  Priority=1  ExternalReset=level  SampleTime=qc_get_step_size  ICPrevOutput=DiscIntNeverNeededParam  ICPrevScaledInput=DiscIntNeverNeededParam
  Logical Operator : Logic  Operator=NOT  AllPortsSameDT=off  OutDataTypeStr=boolean
  Relational Operator : RelationalOperator  InputSameDT=off
  Relational Operator1 : RelationalOperator  InputSameDT=off
  elapsed : Outport  VectorParamsAs1DForOutWhenUnconnected=off
  time : Outport  Port=2  VectorParamsAs1DForOutWhenUnconnected=off
  wires:
  Data Type Conversion/1 -> Discrete-Time Integrator/1
  Signal/1 -> Relational Operator/1
  Threshold/1 -> Relational Operator/2
  Relational Operator/1 -> Data Type Conversion/1, Logical Operator/1
  Logical Operator/1 -> Discrete-Time Integrator/2
  Discrete-Time Integrator/1 -> Relational Operator1/1, time/1
  Duration/1 -> Relational Operator1/2
  Relational Operator1/1 -> elapsed/1

== system Smart_City_QCar2_self_driving_stack/Speed & Steering Commander/Steering Based on LiDAR/Direction Vector Generator ==
  xy_command : Inport
  xy : Inport  Port=2
  heading : Inport  Port=3
  Demux : Demux  Outputs=2
  Display2 : Display  Commented=on
      settings: Decimation=100
  Display5 : Display  Commented=on
      settings: Decimation=100
  Display8 : Display  Commented=on
      settings: Decimation=100
  Radians to Degrees1 : simulink_extras/Transformations/Radians to Degrees
  Radians to Degrees3 : simulink_extras/Transformations/Radians to Degrees
  Signed Sqrt : Sqrt
  Square : Math  Operator=square
  Sum : Sum  Inputs=+-
  Sum1 : Sum  Inputs=+
  Sum3 : Sum  Inputs=+-
  Trigonometric Function : Trigonometry  Operator=atan2
  distance : Outport
  aoa : Outport  Port=2
  wires:
  heading/1 -> Sum3/2
  Sum/1 -> Demux/1, Square/1
  Radians to Degrees3/1 -> Display2/1
  Radians to Degrees1/1 -> Display5/1
  Demux/2 -> Trigonometric Function/1
  Sum1/1 -> Signed Sqrt/1
  Sum3/1 -> aoa/1, Radians to Degrees3/1
  xy/1 -> Sum/2
  Signed Sqrt/1 -> distance/1, Display8/1
  Square/1 -> Sum1/1
  Trigonometric Function/1 -> Radians to Degrees1/1, Sum3/1
  Demux/1 -> Trigonometric Function/2
  xy_command/1 -> Sum/1

== system Smart_City_QCar2_self_driving_stack/Speed & Steering Commander/Traffic Zone 1/Greater Than Threshold ==
  Signal : Inport
  Threshold : Inport  Port=2
  Duration : Inport  Port=3
  Data Type Conversion : DataTypeConversion  SaturateOnIntegerOverflow=off  RndMeth=Floor
  Discrete-Time Integrator : DiscreteIntegrator  Priority=1  ExternalReset=level  SampleTime=qc_get_step_size  ICPrevOutput=DiscIntNeverNeededParam  ICPrevScaledInput=DiscIntNeverNeededParam
  Logical Operator : Logic  Operator=NOT  AllPortsSameDT=off  OutDataTypeStr=boolean
  Relational Operator : RelationalOperator  InputSameDT=off
  Relational Operator1 : RelationalOperator  InputSameDT=off
  elapsed : Outport  VectorParamsAs1DForOutWhenUnconnected=off
  time : Outport  Port=2  VectorParamsAs1DForOutWhenUnconnected=off
  wires:
  Data Type Conversion/1 -> Discrete-Time Integrator/1
  Signal/1 -> Relational Operator/1
  Threshold/1 -> Relational Operator/2
  Relational Operator/1 -> Data Type Conversion/1, Logical Operator/1
  Logical Operator/1 -> Discrete-Time Integrator/2
  Discrete-Time Integrator/1 -> Relational Operator1/1, time/1
  Duration/1 -> Relational Operator1/2
  Relational Operator1/1 -> elapsed/1

== system Smart_City_QCar2_self_driving_stack/Speed & Steering Commander/Traffic Zone 1/Less Than Threshold ==
  Signal : Inport
  Threshold : Inport  Port=2
  Duration : Inport  Port=3
  Data Type Conversion : DataTypeConversion  SaturateOnIntegerOverflow=off  RndMeth=Floor
  Discrete-Time Integrator : DiscreteIntegrator  Priority=1  ExternalReset=level  SampleTime=qc_get_step_size  ICPrevOutput=DiscIntNeverNeededParam  ICPrevScaledInput=DiscIntNeverNeededParam
  Logical Operator : Logic  Operator=NOT  AllPortsSameDT=off  OutDataTypeStr=boolean
  Relational Operator : RelationalOperator  Operator=<  InputSameDT=off
  Relational Operator1 : RelationalOperator  InputSameDT=off
  elapsed : Outport  VectorParamsAs1DForOutWhenUnconnected=off
  time : Outport  Port=2  VectorParamsAs1DForOutWhenUnconnected=off
  wires:
  Relational Operator1/1 -> elapsed/1
  Duration/1 -> Relational Operator1/2
  Discrete-Time Integrator/1 -> time/1, Relational Operator1/1
  Logical Operator/1 -> Discrete-Time Integrator/2
  Relational Operator/1 -> Logical Operator/1, Data Type Conversion/1
  Threshold/1 -> Relational Operator/2
  Signal/1 -> Relational Operator/1
  Data Type Conversion/1 -> Discrete-Time Integrator/1

== system Smart_City_QCar2_self_driving_stack/Speed & Steering Commander/Traffic Zone 2/Greater Than Threshold ==
  Signal : Inport
  Threshold : Inport  Port=2
  Duration : Inport  Port=3
  Data Type Conversion : DataTypeConversion  SaturateOnIntegerOverflow=off  RndMeth=Floor
  Discrete-Time Integrator : DiscreteIntegrator  Priority=1  ExternalReset=level  SampleTime=qc_get_step_size  ICPrevOutput=DiscIntNeverNeededParam  ICPrevScaledInput=DiscIntNeverNeededParam
  Logical Operator : Logic  Operator=NOT  AllPortsSameDT=off  OutDataTypeStr=boolean
  Relational Operator : RelationalOperator  InputSameDT=off
  Relational Operator1 : RelationalOperator  InputSameDT=off
  elapsed : Outport  VectorParamsAs1DForOutWhenUnconnected=off
  time : Outport  Port=2  VectorParamsAs1DForOutWhenUnconnected=off
  wires:
  Relational Operator1/1 -> elapsed/1
  Duration/1 -> Relational Operator1/2
  Discrete-Time Integrator/1 -> time/1, Relational Operator1/1
  Logical Operator/1 -> Discrete-Time Integrator/2
  Relational Operator/1 -> Logical Operator/1, Data Type Conversion/1
  Threshold/1 -> Relational Operator/2
  Signal/1 -> Relational Operator/1
  Data Type Conversion/1 -> Discrete-Time Integrator/1

== system Smart_City_QCar2_self_driving_stack/Speed & Steering Commander/Traffic Zone 2/Less Than Threshold ==
  Signal : Inport
  Threshold : Inport  Port=2
  Duration : Inport  Port=3
  Data Type Conversion : DataTypeConversion  SaturateOnIntegerOverflow=off  RndMeth=Floor
  Discrete-Time Integrator : DiscreteIntegrator  Priority=1  ExternalReset=level  SampleTime=qc_get_step_size  ICPrevOutput=DiscIntNeverNeededParam  ICPrevScaledInput=DiscIntNeverNeededParam
  Logical Operator : Logic  Operator=NOT  AllPortsSameDT=off  OutDataTypeStr=boolean
  Relational Operator : RelationalOperator  Operator=<  InputSameDT=off
  Relational Operator1 : RelationalOperator  InputSameDT=off
  elapsed : Outport  VectorParamsAs1DForOutWhenUnconnected=off
  time : Outport  Port=2  VectorParamsAs1DForOutWhenUnconnected=off
  wires:
  Data Type Conversion/1 -> Discrete-Time Integrator/1
  Signal/1 -> Relational Operator/1
  Threshold/1 -> Relational Operator/2
  Relational Operator/1 -> Data Type Conversion/1, Logical Operator/1
  Logical Operator/1 -> Discrete-Time Integrator/2
  Discrete-Time Integrator/1 -> Relational Operator1/1, time/1
  Duration/1 -> Relational Operator1/2
  Relational Operator1/1 -> elapsed/1

== system Smart_City_QCar2_self_driving_stack/QCar 2/LiDAR/rising edge latch/Latch Input ==
  Input : Inport
  Trigger : TriggerPort  VariantControl=(inherit)
  Constant : Constant
  Latch : Outport  VectorParamsAs1DForOutWhenUnconnected=off
  Executed : Outport  Port=2  VectorParamsAs1DForOutWhenUnconnected=off
  wires:
  Constant/1 -> Executed/1
  Input/1 -> Latch/1
